simulink model "Kubon_lab8_sim"  (R2020b)
settings: Solver=VariableStepAuto  StartTime=0.0  StopTime=10.0  RelTol=1e-3
values from neighbouring files (symbols this model uses):
  A = [ (-cpN*ppN*fk0-ks1-k0)/(Cv1) , k0/Cv1 ; (k0+cpN*ppN*fk0)/(Cv2) , (-k0-cpN*ppN*fk0-ks2)/(Cv2)  ]    [Kubon_lab10.m]    (also in Kubon_lab8.m = [-a1/A1 , a1/A1 ; a1/A2 , (-a1-a2)/A2])
  B = [(cpN*ppN*fk0)/(Cv1) , ks2/Cv1 ; 0 , ks2/Cv2 ]    [Kubon_lab10.m]    (also in Kubon_lab8.m = [1/A1 , 0 ; 0 , 1/A2])
  C = eye(2)    [Kubon_lab10.m]    (also in Kubon_lab8.m)
  D = zeros(2)    [Kubon_lab10.m]    (also in Kubon_lab8.m)
  x0 = 0    [Kubon_lab4.m]    (also in Kubon_lab5.m; Kubon_lab8.m = [h10,h20])
settings Model: Creator=pkubo  LastModifiedBy=pkubo

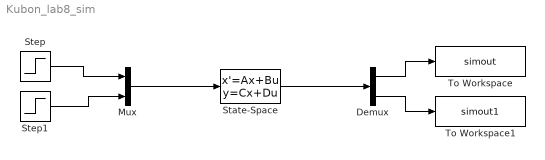
== system Kubon_lab8_sim ==
  Demux : Demux  Outputs=2
  Mux : Mux  Inputs=2
  State-Space : StateSpace  A=A  B=B  C=C  D=D  InitialCondition=x0
  Step : Step  SampleTime=0
  Step1 : Step  SampleTime=0
  To Workspace : ToWorkspace  VariableName=simout  SaveFormat=Timeseries  SampleTime=-1
  To Workspace1 : ToWorkspace  VariableName=simout1  SaveFormat=Timeseries  SampleTime=-1
  wires:
  Mux/1 -> State-Space/1
  State-Space/1 -> Demux/1
  Step/1 -> Mux/1
  Step1/1 -> Mux/2
  Demux/1 -> To Workspace/1
  Demux/2 -> To Workspace1/1
